simulink model "rtwdemo_nestedstructure"  (Simulink 7.1)
settings: Solver=FixedStepDiscrete  StartTime=0.0  StopTime=10.0  RelTol=1e-3
PostLoadFcn:
  | load busobjs.mat
settings Model: Creator=ajayaram  LastModifiedBy=ajayaram
settings OptimizationCC: InlineParams=on  OptimizeModelRefInitCode=on  LifeSpan=1
settings RTWCC: SystemTargetFile=ert.tlc  GenCodeOnly=on  GenerateMakefile=off  TemplateMakefile=ert_default_tmf  Description=Real-Time Workshop Embedded Coder (no auto configuration)  GenerateReport=on  ProcessScript=ert_make_rtw_hook  IncludeHyperlinkInReport=on  LaunchReport=on
settings CodeAppCC: IgnoreCustomStorageClasses=off
settings ERTTargetCC: GenerateSampleERTMain=on  InlinedParameterPlacement=NonHierarchical  RootIOFormat=Structure reference  ERTCustomFileTemplate=example_file_process.tlc

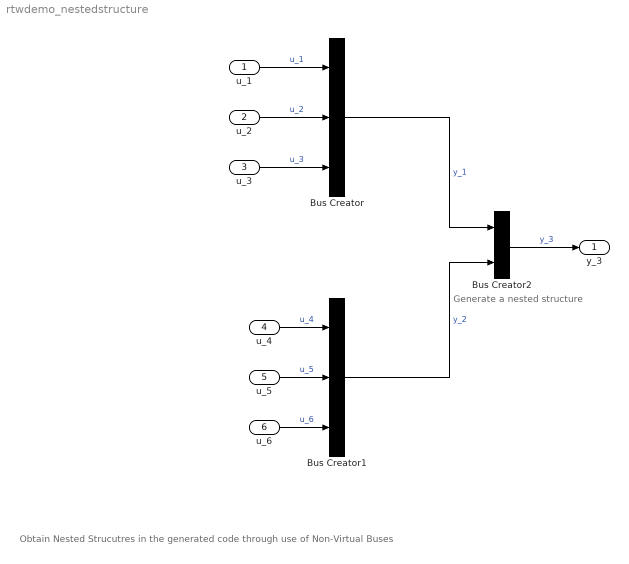
== system rtwdemo_nestedstructure ==
  note: Generate a
      | nested structure
  note: Obtain Nested Strucutres in the generated code
      | through use of Non-Virtual Buses
  u_1 : Inport  OutDataType=sfix(16)  OutScaling=2^0
  u_2 : Inport  Port=2  OutDataType=sfix(16)  OutScaling=2^0
  u_3 : Inport  Port=3  OutDataType=sfix(16)  OutScaling=2^0
  u_4 : Inport  Port=4  OutDataType=sfix(16)  OutScaling=2^0
  u_5 : Inport  Port=5  OutDataType=sfix(16)  OutScaling=2^0
  u_6 : Inport  Port=6  OutDataType=sfix(16)  OutScaling=2^0
  Bus Creator : BusCreator  Inputs=3  UseBusObject=on  NonVirtualBus=on
      settings: BusObject=My_Signals_123
  Bus Creator1 : BusCreator  Inputs=3  UseBusObject=on  NonVirtualBus=on
      settings: BusObject=My_Signals_456
  Bus Creator2 : BusCreator  Inputs=2  UseBusObject=on  NonVirtualBus=on
      settings: BusObject=Nested_Signals
  y_3 : Outport  OutDataType=sfix(16)  OutScaling=2^0
  wires:
  u_1/1 -> Bus Creator/1  "u_1"
  u_2/1 -> Bus Creator/2  "u_2"
  u_3/1 -> Bus Creator/3  "u_3"
  Bus Creator/1 -> Bus Creator2/1  "y_1"
  u_4/1 -> Bus Creator1/1  "u_4"
  u_5/1 -> Bus Creator1/2  "u_5"
  u_6/1 -> Bus Creator1/3  "u_6"
  Bus Creator1/1 -> Bus Creator2/2  "y_2"
  Bus Creator2/1 -> y_3/1  "y_3"
